simulink library "dspswit2"  (Simulink 3.00)
undefined symbols (not defined in the file or in its folder): Low, magnitude
libraries: dspbuff2 x2, dspswit2 x2, dspbdsp2 x1
settings Model: RequirementInfo=9  Creator=don  LastModifiedBy=jeff

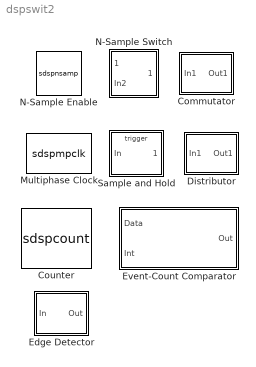
== system dspswit2 ==
  Commutator : Subsystem  mask(Commutator){}
      mask help: Convert a vector into a sequence of scalars produced at a rate N times the input sample rate.
      mask init:
      | S=12; t=(0:S)/S*2*pi; a=0.05; xc=a*cos(t); yc=a*sin(t);
      | xc4=[xc+.45 NaN xc+.35 NaN xc+.45 NaN xc+.8];
      | yc4=[yc+.7 NaN yc+.5 NaN yc+.3 NaN yc+.5];
      | x=[0 .1 NaN .1 .1 .2 .2 .1 NaN .2 .4 NaN .2 .3 NaN .2 .4 NaN .85 1 NaN .75 .525 NaN .595 .525 .55];
      | y=[.5 .5 NaN .2 .8 .8 .2 .2 NaN .7 .7 NaN .5 .5 NaN .3 .3 NaN .5 .5 NaN .5 .7 NaN .7 .7 .61];
      | xs=[xc(4:9) xc(9)+[-.03 0 -.01] ]*3.5+.8;
      | ys=[yc(4:9) yc(9)+[0.01 0 .03 ] ]*3.5+.5;
      mask Help: web(dspbhelp);
      mask Display: plot(xc4,yc4,x,y,xs,ys);
  Counter : S-Function  FunctionName=sdspcount  Parameters=Direction, CountEvent, CounterSize, MaxCount, InitialCount, Output, HitValue, ResetInput, Framebased, SamplesPerFrame, Ts  PortCounts=[]  SFunctionModules=''  mask(Counter){Direction=Down, CountEvent=Rising edge, CounterSize=User defined, MaxCount=255, InitialCount=0, Output=Count and Hit, HitValue=32, ResetInput=on, Framebased=off, SamplesPerFrame=1, Ts=1}
      mask prompts: Direction "Count direction:"; CountEvent "Count event:"; CounterSize "Counter size:"; MaxCount "Maximum count:"; InitialCount "Initial count:"; HitValue "Hit value:"; ResetInput "Reset input"; Framebased "Frame-based clock input"; SamplesPerFrame "Samples per output frame"; Ts "Sample time:"
      mask help: Count up or down based on input count events. If the "Count event" is set to "Free running" the output updates at the specified sample time.
      mask init:
      | [p,xy] = dspblkcount('icon');
      mask Help: web(dspbhelp);
      mask StyleString: popup(Up|Down),popup(Rising edge|Falling edge|Either edge|Non-zero sample|Free running),popup(8 bits|16 bits|32 bits|User defined),edit,edit,popup(Count|Hit|Count and Hit),edit,checkbox,checkbox,edit,edit
      mask CallbackString: |dspblkcount|dspblkcount|||dspblkcount|||||
      mask Display:
      | port_label(p.in1,   p.i1,  p.i1s);
      | port_label(p.in2,   p.i2,  p.i2s);
      | port_label(p.out, p.o1, p.o1s);
      | port_label(p.out, p.o2, p.o2s);
      | disp(xy.direction)
  Distributor : Subsystem  mask(Distributor){N=64, ic=0}
      mask prompts: N "Output vector width, N:"; ic "Initial conditions:"
      mask help: Take scalar input samples and "distribute" them to N outputs (produced as a single vector), reducing the data rate by a factor of N.
      mask init: same as dspswit2/Commutator
      mask Help: web(dspbhelp);
      mask Display: plot(1-xc4,yc4,1-x,y,1-xs,ys);
  Edge Detector : Subsystem  mask(Edge Detector){frame=off, NumChans=1}
      mask prompts: frame "Frame-based inputs"; NumChans "Number of channels:"
      mask help: Output a unity amplitude pulse for one time step in response to a transition from zero to a non-zero value.
      mask init:
      | [x,y] = dspblkedetect('icon');
      | dspblkedetect('update');
      mask Help: web(dspbhelp);
      mask CallbackString: dspblkedetect|
      mask Display: plot(x,y)
  Event-Count Comparator : Subsystem  mask(Event-Count Comparator){Threshold=10}
      mask prompts: Threshold "Event threshold:"
      mask help: Output is true if the number of non-zero inputs over time equals or exceeds the Event threshold during the enable interval. A non-zero input on the interval port (Int) enables the block to begin counting and resets the output. Inputs must be discrete-time.
      mask init:
      | if isempty(Threshold), s=&1; else s=num2str(Threshold); end
      mask Help: web(dspbhelp);
      mask Display:
      | disp('Event-Count\nComparator')
      | text(0.95,0.1,['Thresh:' s],'horiz','right')
  Multiphase Clock : S-Function  FunctionName=sdspmpclk  Parameters=ClkFreq, NumPhases, ActiveLevel, DutyCycle, StartPhase  PortCounts=[]  SFunctionModules=''  mask(Multiphase Clock){ClkFreq=1, NumPhases=4, StartPhase=1, DutyCycle=3, ActiveLevel=High (1)}
      mask prompts: ClkFreq "Clock frequency (Hz):"; NumPhases "Number of phases, N:"; StartPhase "Starting phase (1 to N):"; DutyCycle "Number of phase intervals over which clock is active (1 to N-1):"; ActiveLevel "Active level (polarity):"
      mask help: Generate a vector of N binary signals representing the N clock phases.
      mask init:
      | if isempty(NumPhases), s=&2;
      | else s=num2str(NumPhases);
      | end
      | s=[s '-Phase\nClock'];
      mask Help: web(dspbhelp);
      mask StyleString: edit,edit,edit,edit,popup(High (1)|Low (0))
      mask Display: disp(s)
  N-Sample Enable : S-Function  FunctionName=sdspnsamp  Parameters=TriggerTypeo, N, Ts, ActiveLevel  PortCounts=[]  SFunctionModules=''  mask(N-Sample Enable){N=8, ActiveLevel=Low (0), reset=off, TriggerType=rising, Ts=1}
      mask prompts: N "Trigger count, N:"; ActiveLevel "Active level:"; reset "Reset input"; TriggerType "Trigger type:"; Ts "Sample time:"
      mask help: Transition from inactive to active after the first N samples.
      mask init:
      | [s,x,y, p] = dspblknsample('icon', N, &1);
      | TriggerTypeo = dspblknsample('update', TriggerType);
      mask Help: web(dspbhelp);
      mask StyleString: edit,popup(High (1)|Low (0)),checkbox,popup(rising|falling|either),edit
      mask CallbackString: ||dspblknsample|dspblknsample|
      mask Display:
      | plot(x,y);
      | text(1, 0.05, s,'horiz','right','vert','base');
      | port_label(p.side,p.port,p.label);
  N-Sample Switch : Subsystem  mask(N-Sample Switch){N=8, reset=off, TriggerType=rising, Ts=0.1}
      mask prompts: N "Switch count, N:"; reset "Reset input"; TriggerType "Trigger type:"; Ts "Sample time:"
      mask help: Output N samples from the top port. Thereafter, output samples from the bottom port.
      mask init:
      | [s, x,y] = dspblknswit('icon',N,&1);
      | dspblknswit('update');
      mask Help: web(dspbhelp);
      mask StyleString: edit,checkbox,popup(rising|falling|either),edit
      mask CallbackString: |dspblknswit||
      mask Display:
      | plot(x,y);
      | text(1, 0.05, s,'horiz','right','vert','base');
  Sample and Hold : Subsystem  TreatAsAtomicUnit=on  mask(Sample and Hold){trig=Rising edge, initCond=0}
      mask prompts: trig "Trigger type:"; initCond "Initial condition:"
      mask help: Sample and hold input signal.
      mask init:
      | switch trig
      | case 1, s='rising';
      | case 2, s='falling';
      | case 3, s='either';
      | end
      | set_param([gcb '/Trigger'],'triggertype',s);
      mask Help: web(dspbhelp);
      mask StyleString: popup(Rising edge|Falling edge|Either edge),edit
      mask Display: disp('S/H')

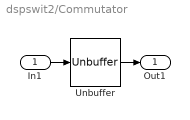
== system dspswit2/Commutator ==
  In1 : Inport  Port=1
  Unbuffer : dspbuff2/Unbuffer  ic=0  num_chans=1
  Out1 : Outport  Port=1  InitialOutput=0
  wires:
  Unbuffer/1 -> Out1/1
  In1/1 -> Unbuffer/1

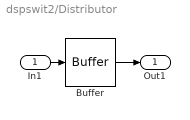
== system dspswit2/Distributor ==
  In1 : Inport  Port=1
  Buffer : dspbuff2/Buffer  N=N  V=0  ic=ic
  Out1 : Outport  Port=1  InitialOutput=0
  wires:
  In1/1 -> Buffer/1
  Buffer/1 -> Out1/1

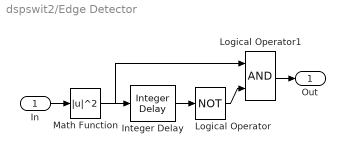
== system dspswit2/Edge Detector ==
  In : Inport  Port=1
  Integer Delay : dspbdsp2/Integer Delay  delay=1  ic=1  frame=off  df=on  numChans=NumChans
  Logical Operator : Logic  Operator=NOT  Inputs=1
  Logical Operator1 : Logic  Operator=AND  Inputs=2
  Math Function : Math  Operator=magnitude^2  OutputSignalType=auto
  Out : Outport  Port=1  InitialOutput=0
  wires:
  Integer Delay/1 -> Logical Operator/1
  Logical Operator/1 -> Logical Operator1/2
  Logical Operator1/1 -> Out/1
  In/1 -> Math Function/1
  Math Function/1 -> Integer Delay/1, Logical Operator1/1

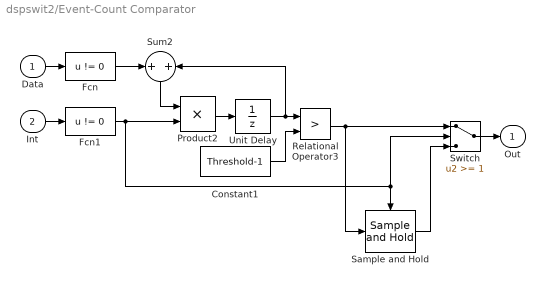
== system dspswit2/Event-Count Comparator ==
  Data : Inport  Port=1
  Int : Inport  Port=2
  Constant1 : Constant  Value=Threshold-1
  Fcn : Fcn  Expr=u != 0
  Fcn1 : Fcn  Expr=u != 0
  Product2 : Product  Inputs=2  Multiplication=Element-wise(.*)  SaturateOnIntegerOverflow=on
  Relational Operator3 : RelationalOperator  Operator=>
  Sample and Hold : dspswit2/Sample and Hold  trig=Falling edge  initCond=0
  Sum2 : Sum  Orientation=down  Inputs=+|+  SaturateOnIntegerOverflow=on
  Switch : Switch  Threshold=1
  Unit Delay : UnitDelay  X0=0  SampleTime=-1
  Out : Outport  Port=1
  wires:
  Sample and Hold/1 -> Switch/3
  Relational Operator3/1 -> Switch/1, Sample and Hold/1
  Switch/1 -> Out/1
  Fcn1/1 -> Switch/2, Sample and Hold/Trigger, Product2/2
  Sum2/1 -> Product2/1
  Product2/1 -> Unit Delay/1
  Unit Delay/1 -> Relational Operator3/1, Sum2/2
  Constant1/1 -> Relational Operator3/2
  Data/1 -> Fcn/1
  Fcn/1 -> Sum2/1
  Int/1 -> Fcn1/1

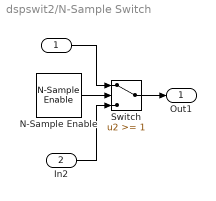
== system dspswit2/N-Sample Switch ==
  " " : Inport  Port=1
  In2 : Inport  Port=2
  N-Sample Enable : dspswit2/N-Sample Enable  N=N  ActiveLevel=Low (0)  reset=off  TriggerType=rising  Ts=Ts
  Switch : Switch  Threshold=1
  Out1 : Outport  Port=1
  wires:
  N-Sample Enable/1 -> Switch/2
  Switch/1 -> Out1/1
  " "/1 -> Switch/1
  In2/1 -> Switch/3

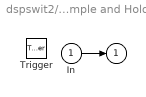
== system dspswit2/Sample and Hold ==
  In : Inport  Port=1
  Trigger : TriggerPort  TriggerType=rising  OutputDataType=auto
  " " : Outport  Port=1  InitialOutput=initCond
  wires:
  In/1 -> " "/1
